simulink model "parte4_eje1_Thidraulica_NoLineal"  (R2019b)
settings: Solver=VariableStepAuto  StartTime=0.0  StopTime=10.0  RelTol=1e-3
values from neighbouring files (symbols this model uses):
  At = 1/(gFL-gNL)    (= 1.25)    [parte4_ej1_ThidraulicaNLdata.m]    (also in parte4_eje2_Thidraulica_const.m)
  Ho = 1    [parte4_ej1_ThidraulicaNLdata.m]    (also in parte4_eje2_Thidraulica_const.m)
  Pr = 1.274    [parte4_ej1_ThidraulicaNLdata.m]
  TW = 1    [parte4_ej1_ThidraulicaNLdata.m]    (also in parte4_eje2_Thidraulica_const.m)
  UNL = 0.068    [parte4_ej1_ThidraulicaNLdata.m]    (also in parte4_eje2_Thidraulica_const.m = 0.08)
  w = 1    [parte4_ej1_ThidraulicaNLdata.m]    (also in parte4_eje2_Thidraulica_const.m)
settings Model: Creator=cjuar  LastModifiedBy=cjuar

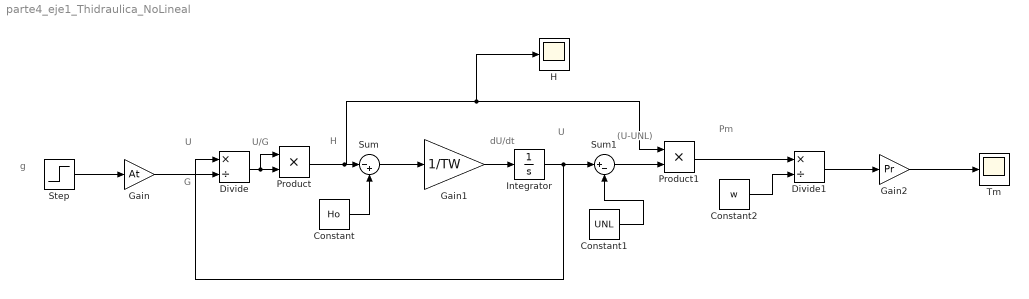
== system parte4_eje1_Thidraulica_NoLineal ==
  note: Pm
  note: (U-UNL)
  note: H
  note: U/G
  note: U
  note: G
  note: U
  note: dU/dt
  note: g
  Constant : Constant  Value=Ho
  Constant1 : Constant  Value=UNL
  Constant2 : Constant  Value=w
  Divide : Product  Inputs=*/
  Divide1 : Product  Inputs=*/
  Gain : Gain  Gain=At
  Gain1 : Gain  Gain=1/TW
  Gain2 : Gain  Gain=Pr
  H : Scope
  Integrator : Integrator
  Product : Product
  Product1 : Product
  Step : Step  Time=0.8  Before=0.001  SampleTime=0
  Sum : Sum  Inputs=|-+
  Sum1 : Sum  Inputs=|+-
  Tm : Scope
  wires:
  Gain1/1 -> Integrator/1
  Integrator/1 -> Divide/1, Sum1/1
  Gain/1 -> Divide/2
  Divide/1 -> Product/1, Product/2
  Product/1 -> H/1, Product1/1, Sum/1
  Constant/1 -> Sum/2
  Sum/1 -> Gain1/1
  Constant1/1 -> Sum1/2
  Sum1/1 -> Product1/2
  Product1/1 -> Divide1/1
  Constant2/1 -> Divide1/2
  Divide1/1 -> Gain2/1
  Gain2/1 -> Tm/1
  Step/1 -> Gain/1
